simulink model "horizontales_drehungsfreies_Windfeld"  (R2020b)
settings: Solver=VariableStepAuto  StartTime=0.0  StopTime=10.0  RelTol=1e-3
settings Model: Creator=Dogukan  LastModifiedBy=Dogukan

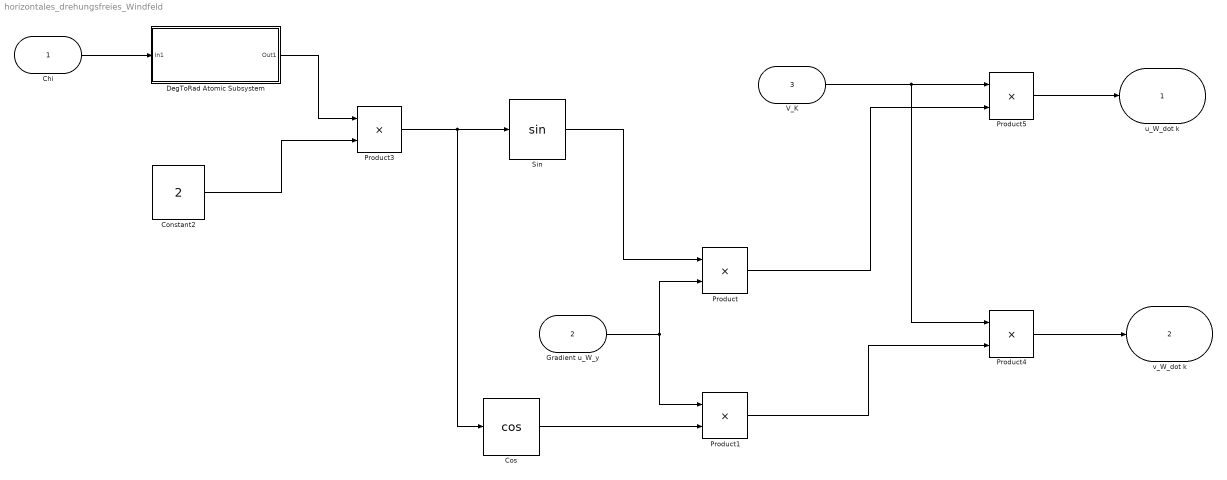
== system horizontales_drehungsfreies_Windfeld ==
  Chi : Inport
  Gradient u_W_y : Inport  Port=2
  V_K : Inport  Port=3
  Constant2 : Constant  Value=2
  Cos : Trigonometry  Operator=cos
  DegToRad Atomic Subsystem : Subsystem  TreatAsAtomicUnit=on
  Product{,1,3..5} (5 alike) : Product
  Sin : Trigonometry
  u_W_dot k : Outport
  v_W_dot k : Outport  Port=2
  wires:
  Chi/1 -> DegToRad Atomic Subsystem/1(In1)
  Constant2/1 -> Product3/2
  DegToRad Atomic Subsystem/1(Out1) -> Product3/1
  Product3/1 -> Cos/1, Sin/1
  Sin/1 -> Product/1
  Gradient u_W_y/1 -> Product/2, Product1/1
  Product/1 -> Product5/2
  Product5/1 -> u_W_dot k/1
  V_K/1 -> Product4/1, Product5/1
  Product1/1 -> Product4/2
  Product4/1 -> v_W_dot k/1
  Cos/1 -> Product1/2

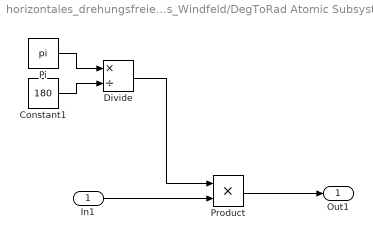
== system horizontales_drehungsfreies_Windfeld/DegToRad Atomic Subsystem ==
  In1 : Inport
  Constant1 : Constant  Value=180
  Divide : Product  Inputs=*/
  Pi : Constant  Value=pi  OutDataTypeStr=Inherit: Inherit via back propagation
  Product : Product
  Out1 : Outport
  wires:
  Pi/1 -> Divide/1
  Constant1/1 -> Divide/2
  Divide/1 -> Product/1
  In1/1 -> Product/2
  Product/1 -> Out1/1
